simulink model "ideal_buck"  (R2018a)
settings: Solver=VariableStepAuto  StartTime=0.0  StopTime=2  RelTol=1e-3
undefined symbols (not defined in the file): A, B, Co, L, opt_pwm, opt_theorem, P, Q, R, Ro, sys, Ti, Vs, xe
libraries: powerlib x12, simulink x2, pePwmGenerator x1
settings Model: SimulationMode=accelerator  Creator=TARCIO-FEM  LastModifiedBy=julio

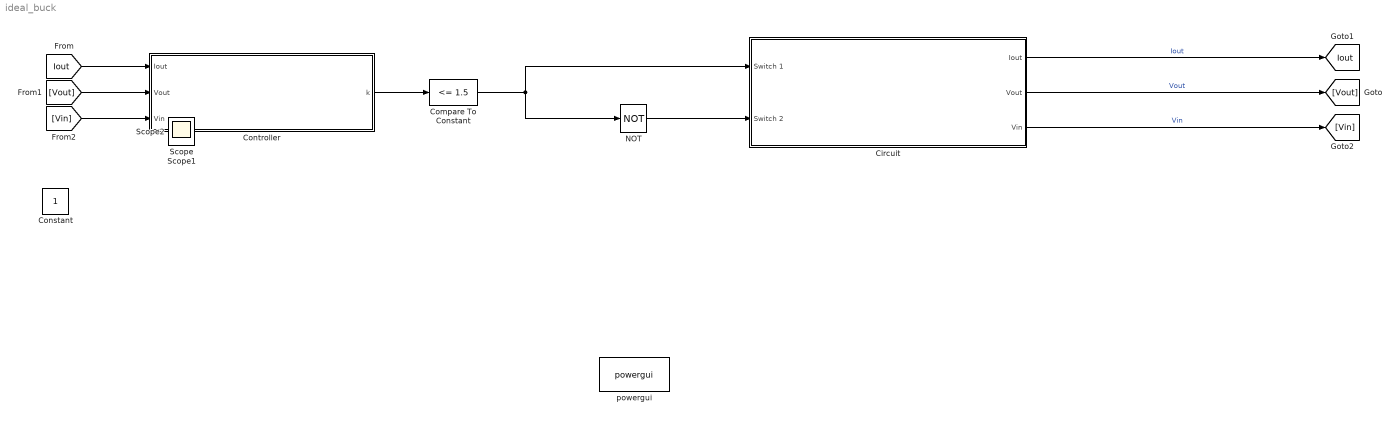
== system ideal_buck ==
  Circuit : Subsystem
  Compare To Constant : simulink/Logic and Bit Operations/Compare To Constant  relop=<=  const=1.5  OutDataTypeStr=boolean
  Controller : Subsystem
  NOT : Logic  Operator=NOT  IconShape=distinctive  AllPortsSameDT=off  OutDataTypeStr=boolean
  powergui : powerlib/powergui  Priority=1  SimulationMode=Discrete  SampleTime=Ti  frequency=60  Iterations=50  frequencyindice=0  Pbase=100e6  ErrMax=1e-4  UnitsV=kV  UnitsW=MW  buscounter=0  FunctionMessages=off  echomessages=off  EnableUseOfTLC=off  CurrentSourceSwitches=off  DisableSnubberDevices=off  DisableRonSwitches=off  DisableVfSwitches=off  DisplayEquations=off  SolverType=Tustin/Backward Euler (TBE)  Interpol=off  ExternalGateDelay=off  methode=off  Ts=100  x0status=blocks  SPID=on  SwTol=0  HookPort=off  RestoreLinks=warning  ResistiveCurrentMeasurement=off  Frange=[0:2:500]  Ylog=off  Xlog=on  ShowGrid=off  save=off  variable=ZData  structure=0  ZoomFFT=off  StartTime=0.0  cycles=1  DisplayStyle=1  fundamental=60  FreqAxis=off  MaxFrequency=1000  frequencyindicesteady=1  RmsSteady=1  display=off
  Constant : Constant  IOType=siggen
  Scope : Scope
  Scope1 : Scope
  Scope2 : Scope
  tag scope: Iout=global
  wires:
  Compare To Constant/1 -> Circuit/1(Switch 1), NOT/1
  NOT/1 -> Circuit/2(Switch 2)
  Circuit/1(Iout) -> [Iout]  "Iout"
  Circuit/2(Vout) -> [Vout]  "Vout"
  Circuit/3(Vin) -> [Vin]  "Vin"
  [Iout] -> Controller/1(Iout)
  [Vout] -> Controller/2(Vout)
  [Vin] -> Controller/3(Vin)
  Controller/1(k) -> Compare To Constant/1

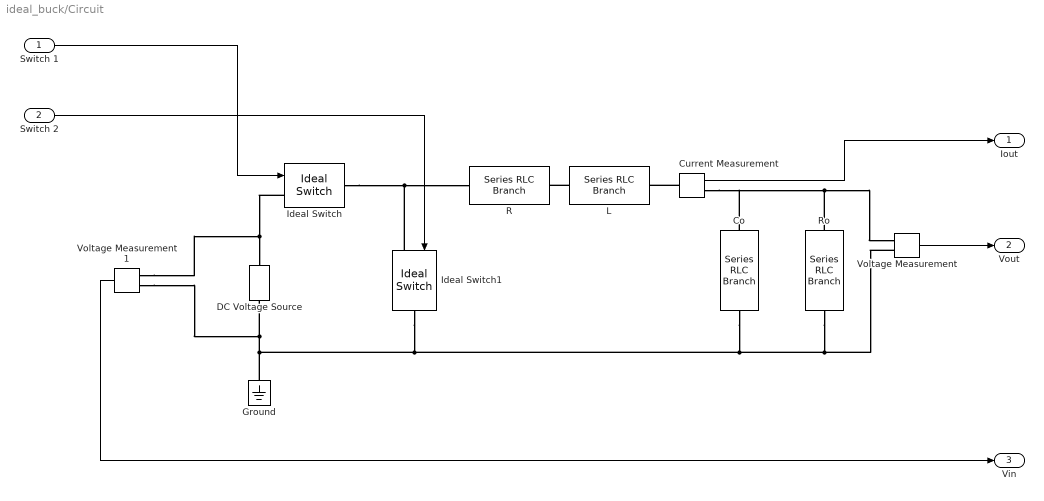
== system ideal_buck/Circuit ==
  Switch 1 : Inport
  Switch 2 : Inport  Port=2
  Co : powerlib/Elements/Series RLC Branch  LConnTagsString=__new0  RConnTagsString=__new0  BranchType=C  Resistance=1  Inductance=L  SetiL0=off  InitialCurrent=0  Capacitance=Co  Setx0=off  InitialVoltage=0  Measurements=None
  Current Measurement : powerlib/Measurements/Current Measurement  PhasorSimulation=off  OutputType=Complex  PSBequivalent=0
  DC Voltage Source : powerlib/Electrical Sources/DC Voltage Source  Amplitude=Vs  Measurements=None
  Ground : powerlib/Elements/Ground  LConnTagsString=a
  Ideal Switch : powerlib/Power Electronics/Ideal Switch  Ron=0.001  Lon=0  IC=0  Rs=1e5  Cs=inf  Measurements=off
  Ideal Switch1 : powerlib/Power Electronics/Ideal Switch  Ron=0.001  Lon=0  IC=0  Rs=1e5  Cs=inf  Measurements=off
  L : powerlib/Elements/Series RLC Branch  LConnTagsString=__new0  RConnTagsString=__new0  BranchType=L  Resistance=1  Inductance=L  SetiL0=off  InitialCurrent=0  Capacitance=1e-6  Setx0=off  InitialVoltage=0  Measurements=None
  R : powerlib/Elements/Series RLC Branch  LConnTagsString=__new0  RConnTagsString=__new0  BranchType=R  Resistance=R  Inductance=1e-3  SetiL0=off  InitialCurrent=0  Capacitance=1e-6  Setx0=off  InitialVoltage=0  Measurements=None
  Ro : powerlib/Elements/Series RLC Branch  LConnTagsString=__new0  RConnTagsString=__new0  BranchType=R  Resistance=Ro  Inductance=1e-3  SetiL0=off  InitialCurrent=0  Capacitance=1e-6  Setx0=off  InitialVoltage=0  Measurements=None
  Voltage Measurement : powerlib/Measurements/Voltage Measurement  PhasorSimulation=off  OutputType=Complex  PSBequivalent=0
  Voltage Measurement1 : powerlib/Measurements/Voltage Measurement  PhasorSimulation=off  OutputType=Complex  PSBequivalent=0
  Iout : Outport
  Vout : Outport  Port=2
  Vin : Outport  Port=3
  wires:
  Switch 1/1 -> Ideal Switch/1
  Voltage Measurement1/1 -> Vin/1
  Current Measurement/1 -> Iout/1
  Voltage Measurement/1 -> Vout/1
  Switch 2/1 -> Ideal Switch1/1
  connections:
  L/LConn1 -- R/RConn1
  Ideal Switch/RConn1 -- Ideal Switch1/LConn1 -- R/LConn1
  Current Measurement/LConn1 -- L/RConn1
  Ideal Switch/LConn1 -- Voltage Measurement1/LConn1 -- DC Voltage Source/RConn1
  Ro/LConn1 -- Voltage Measurement/LConn1 -- Co/LConn1 -- Current Measurement/RConn1
  Ro/RConn1 -- Voltage Measurement/LConn2 -- Co/RConn1 -- Ideal Switch1/RConn1 -- Ground/LConn1 -- Voltage Measurement1/LConn2 -- DC Voltage Source/LConn1

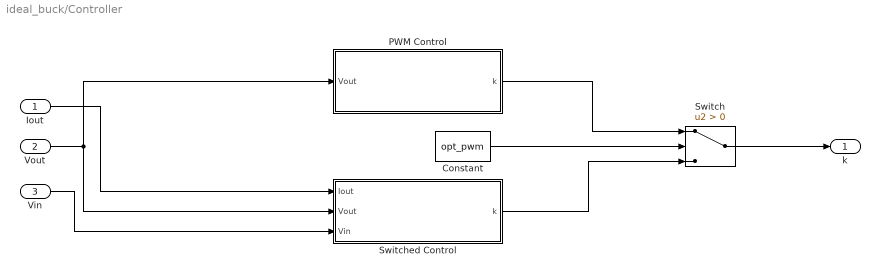
== system ideal_buck/Controller ==
  Iout : Inport
  Vout : Inport  Port=2
  Vin : Inport  Port=3
  Constant : Constant  Value=opt_pwm
  PWM Control : Subsystem
  Switch : Switch  Criteria=u2 > Threshold
  Switched Control : Subsystem
  k : Outport
  wires:
  Iout/1 -> Switched Control/1(Iout)
  Vout/1 -> PWM Control/1(Vout), Switched Control/2(Vout)
  Vin/1 -> Switched Control/3(Vin)
  Switch/1 -> k/1
  PWM Control/1(k) -> Switch/1
  Switched Control/1(k) -> Switch/3
  Constant/1 -> Switch/2

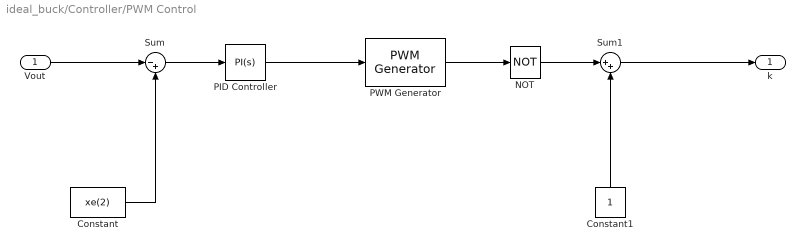
== system ideal_buck/Controller/PWM Control ==
  Vout : Inport
  Constant : Constant  Value=xe(2)
  Constant1 : Constant
  NOT : Logic  Operator=NOT  IconShape=distinctive  AllPortsSameDT=off  OutDataTypeStr=boolean
  PID Controller : simulink/Continuous/PID Controller  Controller=PI  TimeDomain=Continuous-time  SampleTime=-1  IntegratorMethod=Forward Euler  FilterMethod=Forward Euler  Form=Ideal  UseFilter=on  ControllerParametersSource=internal  P=0.05  I=100  D=1  N=100  InitialConditionSource=internal  InitialConditionForIntegrator=0  InitialConditionForFilter=0  ExternalReset=none  LimitOutput=off  UpperSaturationLimit=inf  LowerSaturationLimit=-inf  LinearizeAsGain=on  AntiWindupMode=none  Kb=1  TrackingMode=off  Kt=1  PParamMin=[]  PParamMax=[]  IParamMin=[]  IParamMax=[]  DParamMin=[]  DParamMax=[]  NParamMin=[]  NParamMax=[]  KbParamMin=[]  KbParamMax=[]  KtParamMin=[]  KtParamMax=[]  POutMin=[]  POutMax=[]  IOutMin=[]  IOutMax=[]  DOutMin=[]  DOutMax=[]  NOutMin=[]  NOutMax=[]  KbOutMin=[]  KbOutMax=[]  KtOutMin=[]  KtOutMax=[]  IntegratorOutMin=[]  IntegratorOutMax=[]  FilterOutMin=[]  FilterOutMax=[]  SumOutMin=[]  SumOutMax=[]  SumI1OutMin=[]  SumI1OutMax=[]  SumI2OutMin=[]  SumI2OutMax=[]  SumI3OutMin=[]  SumI3OutMax=[]  SumDOutMin=[]  SumDOutMax=[]  SaturationOutMin=[]  SaturationOutMax=[]  IntegratorContinuousStateAttributes=''  IntegratorStateMustResolveToSignalObject=off  IntegratorRTWStateStorageClass=Auto  FilterContinuousStateAttributes=''  FilterStateMustResolveToSignalObject=off  FilterRTWStateStorageClass=Auto  DifferentiatorICPrevScaledInput=0  DifferentiatorOutMin=[]  DifferentiatorOutMax=[]  FilterDiffOutCoefMin=[]  FilterDiffOutCoefMax=[]  SumDenOutMin=[]  SumDenOutMax=[]  SumNumOutMin=[]  SumNumOutMax=[]  ReciprocalOutMin=[]  ReciprocalOutMax=[]  DivideOutMin=[]  DivideOutMax=[]  TunerSelectOption=Transfer Function Based (PID Tuner App)
  PWM Generator : pePwmGenerator/PWM Generator  CarrCount=Up  Tper=1e-5  Ts=1e-6
  Sum : Sum  Inputs=|-+
  Sum1 : Sum  Inputs=|++
  k : Outport
  wires:
  Vout/1 -> Sum/1
  Sum/1 -> PID Controller/1
  Constant/1 -> Sum/2
  PID Controller/1 -> PWM Generator/1
  Sum1/1 -> k/1
  PWM Generator/1 -> NOT/1
  Constant1/1 -> Sum1/2
  NOT/1 -> Sum1/1

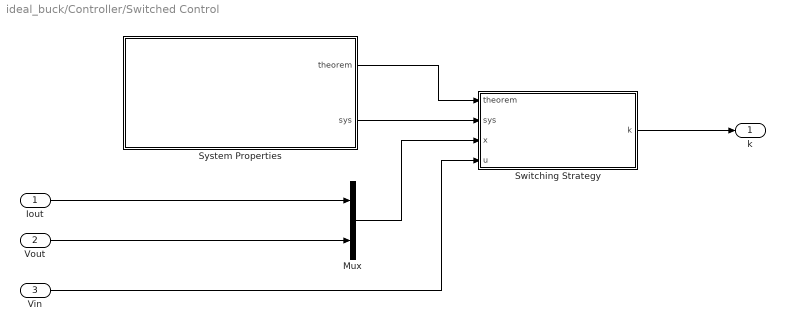
== system ideal_buck/Controller/Switched Control ==
  Iout : Inport
  Vout : Inport  Port=2
  Vin : Inport  Port=3
  Mux : Mux  Inputs=2
  Switching Strategy : MATLAB Function  TreatAsAtomicUnit=on
  System Properties : Subsystem
  k : Outport
  wires:
  Vin/1 -> Switching Strategy/4(u)
  Switching Strategy/1(k) -> k/1
  System Properties/1(theorem) -> Switching Strategy/1(theorem)
  System Properties/2(sys) -> Switching Strategy/2(sys)
  Mux/1 -> Switching Strategy/3(x)
  Iout/1 -> Mux/1
  Vout/1 -> Mux/2

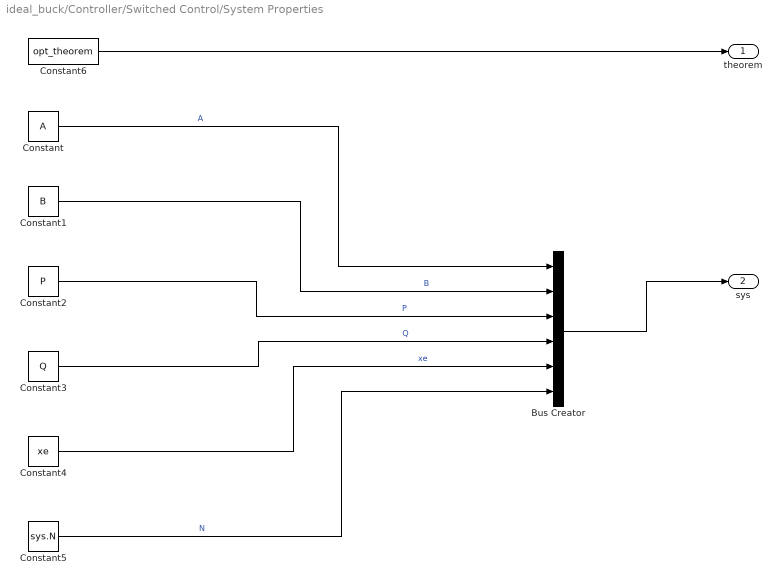
== system ideal_buck/Controller/Switched Control/System Properties ==
  Bus Creator : BusCreator  Inputs=6  OutDataTypeStr=Bus: SystemDataBus
  Constant : Constant  Value=A  VectorParams1D=off
  Constant1 : Constant  Value=B  VectorParams1D=off
  Constant2 : Constant  Value=P  VectorParams1D=off
  Constant3 : Constant  Value=Q  VectorParams1D=off
  Constant4 : Constant  Value=xe  VectorParams1D=off
  Constant5 : Constant  Value=sys.N
  Constant6 : Constant  Value=opt_theorem
  theorem : Outport
  sys : Outport  Port=2
  wires:
  Bus Creator/1 -> sys/1
  Constant2/1 -> Bus Creator/3  "P"
  Constant1/1 -> Bus Creator/2  "B"
  Constant/1 -> Bus Creator/1  "A"
  Constant3/1 -> Bus Creator/4  "Q"
  Constant4/1 -> Bus Creator/5  "xe"
  Constant5/1 -> Bus Creator/6  "N"
  Constant6/1 -> theorem/1

== matlab function ideal_buck/Controller/Switched Control/Switching Strategy ==
  data: theorem input; sys input; x input; u input; k output
function k = switching_strategy(theorem, sys, x, u)
    qsi = x - sys.xe;
    sig = zeros(sys.N,1);
    
    for i=1:sys.N
        switch(theorem)
            case 1
                sig(i) = qsi'*(sys.Q(:,:,i)*qsi + 2*sys.P*(sys.A(:,:,i)*x + sys.B(:,:,i)*u));
            case 2
                sig(i) = qsi'*sys.P*(sys.A(:,:,i)*sys.xe + sys.B(:,:,i)*u);
        end
    end
    [~, k] = min(sig);
end
